simulink model "PI_controller"  (R2020b)
settings: Solver=VariableStepAuto  StartTime=0.0  StopTime=10.0  RelTol=1e-3
settings Model: Creator=saadh  LastModifiedBy=saadh
settings DataIOCC: SaveOutput=off  SaveTime=off

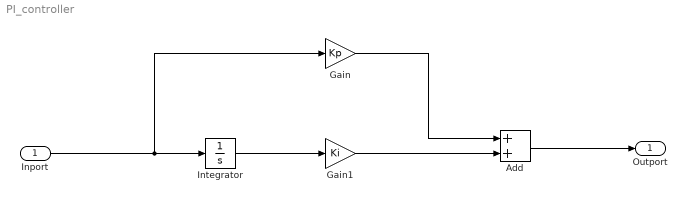
== system PI_controller ==
  Inport : Inport  OutDataTypeStr=double  PortDimensions=1  SampleTime=0
  Add : Sum
  Gain : Gain  Gain=Kp  mask{Kp=800}
  Gain1 : Gain  Gain=Ki  mask{Ki=40}
  Integrator : Integrator
  Outport : Outport  OutDataTypeStr=double  PortDimensions=1  SampleTime=0
  wires:
  Inport/1 -> Integrator/1, Gain/1
  Integrator/1 -> Gain1/1
  Gain1/1 -> Add/2
  Gain/1 -> Add/1
  Add/1 -> Outport/1
